simulink model "conv_AM_system"  (R2019b)
settings: Solver=VariableStepAuto  StartTime=0.0  StopTime=1  RelTol=1e-3
libraries: simulink x1, dsparch4 x1, dspsigops x1
settings Model: Creator=SEFA  LastModifiedBy=SEFA

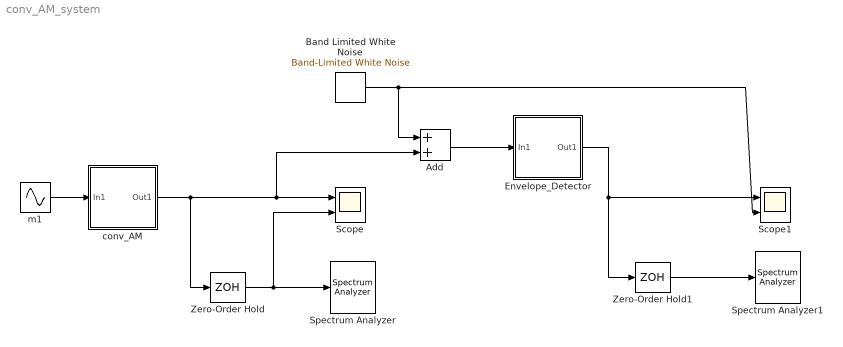
== system conv_AM_system ==
  Add : Sum
  Band Limited White Noise : simulink/Sources/Band-Limited White Noise  Cov=[0]  Ts=1e-5  seed=[23341]
  Envelope_Detector : Subsystem
  Scope : Scope  NumInputPorts=2
  Scope1 : Scope  NumInputPorts=2
  Spectrum Analyzer : SpectrumAnalyzer
  Spectrum Analyzer1 : SpectrumAnalyzer
  Zero-Order Hold : ZeroOrderHold  SampleTime=5e-4
  Zero-Order Hold1 : ZeroOrderHold  SampleTime=5e-4
  conv_AM : Subsystem
  m1 : Sin  Frequency=2*pi*50  Phase=pi/2  SampleTime=1e-5
  wires:
  Zero-Order Hold/1 -> Scope/2, Spectrum Analyzer/1
  m1/1 -> conv_AM/1(In1)
  Envelope_Detector/1(Out1) -> Zero-Order Hold1/1, Scope1/1
  Zero-Order Hold1/1 -> Spectrum Analyzer1/1
  Add/1 -> Envelope_Detector/1(In1)
  conv_AM/1(Out1) -> Zero-Order Hold/1, Add/2, Scope/1
  Band Limited White Noise/1 -> Add/1, Scope1/2

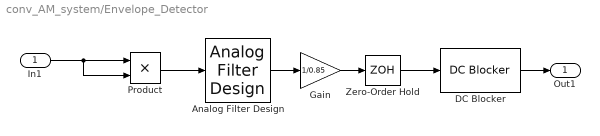
== system conv_AM_system/Envelope_Detector ==
  In1 : Inport
  Analog Filter Design : dsparch4/Analog Filter Design  method=Butterworth  filttype=Lowpass  N=8  Wlo=2*pi*75  Whi=80  Rp=2  Rs=40
  DC Blocker : dspsigops/DC Blocker  Algorithm=IIR  NormalizedBandwidth=0.001  Length=8  Order=6  SimulateUsing=Code generation
      settings: SourceProductName=DSP System Toolbox  SourceProductBaseCode=DS
  Gain : Gain  Gain=1/0.85
  Product : Product
  Zero-Order Hold : ZeroOrderHold  SampleTime=1e-5
  Out1 : Outport
  wires:
  In1/1 -> Product/2, Product/1
  Analog Filter Design/1 -> Gain/1
  DC Blocker/1 -> Out1/1
  Gain/1 -> Zero-Order Hold/1
  Zero-Order Hold/1 -> DC Blocker/1
  Product/1 -> Analog Filter Design/1

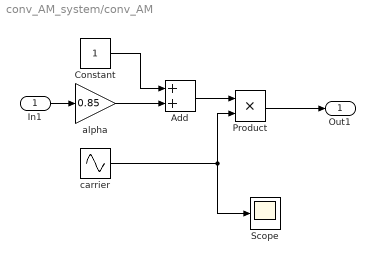
== system conv_AM_system/conv_AM ==
  In1 : Inport
  Add : Sum
  Constant : Constant
  Product : Product
  Scope : Scope
  alpha : Gain  Gain=0.85
  carrier : Sin  Frequency=2*pi*500  Phase=pi/2  SampleTime=1e-5
  Out1 : Outport
  wires:
  carrier/1 -> Product/2, Scope/1
  Product/1 -> Out1/1
  Add/1 -> Product/1
  alpha/1 -> Add/2
  In1/1 -> alpha/1
  Constant/1 -> Add/1
